simulink model "s_aero_2dof_lqr_control"  (R2017a)
settings: Solver=ode1  StartTime=0.0  StopTime=30  FixedStep=0.002  RelTol=1e-3  EnableMultiTasking=on
values from neighbouring files (symbols this model uses):
  K = lqr(A,B,Q,R)    [quanser_aero_lqr.m]    (also in quanser_aero_pd_design.m = Kyy/Dy)
undefined symbols (not defined in the file or in its folder): A, B, C, D
libraries: simulink_extras x4, quarc_library x2
settings Model: ExtModeTrigDuration=5000  Creator=MLevis  LastModifiedBy=Administrator
settings SolverCC: PositivePriorityOrder=on
settings DataIOCC: LimitDataPoints=on  SaveFormat=Array
settings OptimizationCC: LifeSpan=inf
settings DebuggingCC: SolverPrmCheckMsg=warning  SFUnexpectedBacktrackingDiag=warning  SFNoUnconditionalDefaultTransitionDiag=warning  SFExecutionAtInitializationDiag=none
settings HardwareCC: ProdBitPerPointer=32  ProdBitPerSizeT=32  ProdBitPerPtrDiffT=32  ProdLargestAtomicFloat=None  ProdIntDivRoundTo=Undefined  ProdEndianess=Unspecified  ProdWordSize=32  ProdHWDeviceType=32-bit Generic
settings ModelReferenceCC: PropagateSignalLabelsOutOfModel=off
settings RTWCC: SystemTargetFile=quarc_win64.tlc  TemplateMakefile=quarc_default_tmf  Description=QUARC Win64 Target
settings STFCustomTargetCC: TargetPreCompLibLocation=C:\PROGRA~3\QUARC\lib\2014a\win64\release  ConcurrentExecutionCompliant=on  GeneratePreprocessorConditionals=Disable all  SystemTargetFile=quarc_win64.tlc
settings GRTTargetCC: TargetPreCompLibLocation=C:\PROGRA~3\QUARC\lib\2014a\win64\release  TargetLangStandard=C89/C90 (ANSI)  ParMdlRefBuildCompliant=off  CompOptLevelCompliant=off  GeneratePreprocessorConditionals=Disable all  CombineOutputUpdateFcns=off  MatFileLogging=off  CPPClassGenCompliant=off  GRTInterface=on  UseToolchainInfoCompliant=off  ExtMode=on  ExtModeMexFile=quarc_comm
settings ConfigComp: CovMetricSettings=dw  CovHtmlReporting=on  CovSaveCumulativeToWorkspaceVar=on  CovSaveSingleToWorkspaceVar=on  CovExternalEMLEnable=off  CovSFcnEnable=off

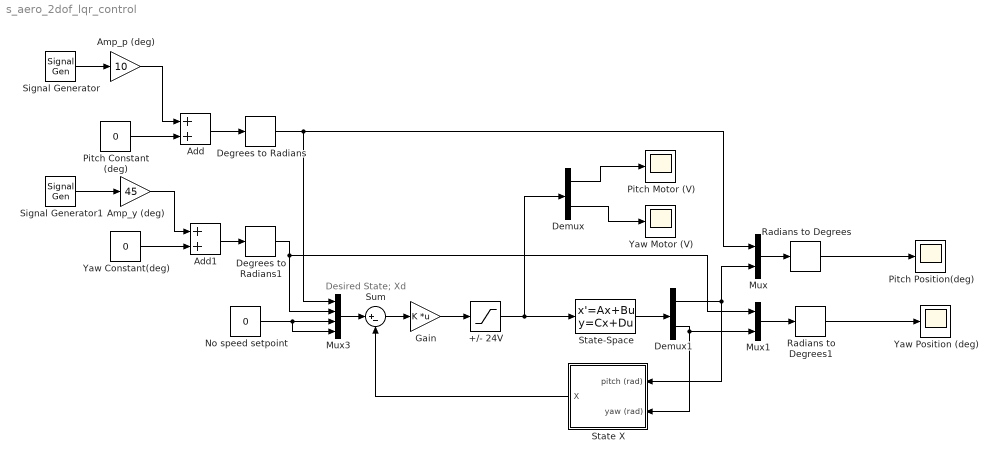
== system s_aero_2dof_lqr_control ==
  note: Desired State; Xd
  +/- 24V : Saturate  UpperLimit=24  LowerLimit=-24
  Add : Sum
  Add1 : Sum
  Amp_p (deg) : Gain  Gain=10
  Amp_y (deg) : Gain  Gain=45
  Degrees to Radians : simulink_extras/Transformations/Degrees to Radians
  Degrees to Radians1 : simulink_extras/Transformations/Degrees to Radians
  Demux : Demux  Outputs=2
  Demux1 : Demux  Outputs=2
  Gain : Gain  Gain=K  Multiplication=Matrix(K*u)
  Mux : Mux  Inputs=2
  Mux1 : Mux  Inputs=2
  Mux3 : Mux
  No speed setpoint : Constant  Value=0
  Pitch Constant (deg) : Constant  Value=0
  Pitch Motor (V) : Scope
  Pitch Position(deg) : Scope
  Radians to Degrees : simulink_extras/Transformations/Radians to Degrees
  Radians to Degrees1 : simulink_extras/Transformations/Radians to Degrees
  Signal Generator : SignalGenerator  WaveForm=square  Frequency=0.1
  Signal Generator1 : SignalGenerator  WaveForm=square  Frequency=0.04
  State X : Subsystem
  State-Space : StateSpace  A=A  B=B  C=C  D=D  X0=0
  Sum : Sum  Inputs=|+-
  Yaw Constant(deg) : Constant  Value=0
  Yaw Motor (V) : Scope
  Yaw Position (deg) : Scope
  wires:
  Degrees to Radians/1 -> Mux3/1, Mux/1
  Degrees to Radians1/1 -> Mux3/2, Mux1/1
  Signal Generator/1 -> Amp_p (deg)/1
  Pitch Constant (deg)/1 -> Add/2
  Add/1 -> Degrees to Radians/1
  Yaw Constant(deg)/1 -> Add1/2
  Amp_p (deg)/1 -> Add/1
  Signal Generator1/1 -> Amp_y (deg)/1
  Amp_y (deg)/1 -> Add1/1
  Add1/1 -> Degrees to Radians1/1
  Mux/1 -> Radians to Degrees/1
  Radians to Degrees/1 -> Pitch Position(deg)/1
  Radians to Degrees1/1 -> Yaw Position (deg)/1
  Gain/1 -> +/- 24V/1
  Demux/1 -> Pitch Motor (V)/1
  Demux/2 -> Yaw Motor (V)/1
  Sum/1 -> Gain/1
  Mux1/1 -> Radians to Degrees1/1
  Mux3/1 -> Sum/1
  No speed setpoint/1 -> Mux3/4, Mux3/3
  +/- 24V/1 -> State-Space/1, Demux/1
  State X/1(X) -> Sum/2
  Demux1/1 -> Mux/2, State X/1(pitch (rad))
  State-Space/1 -> Demux1/1
  Demux1/2 -> Mux1/2, State X/2(yaw (rad))

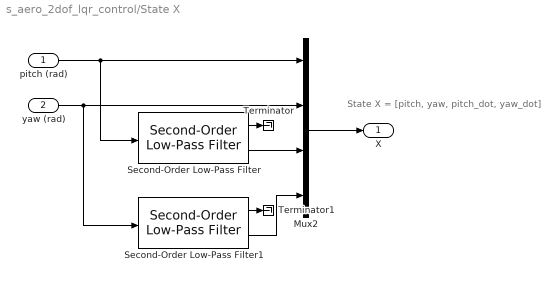
== system s_aero_2dof_lqr_control/State X ==
  note: State X = [pitch, yaw, pitch_dot, yaw_dot]
  pitch (rad) : Inport
  yaw (rad) : Inport  Port=2
  Mux2 : Mux
  Second-Order Low-Pass Filter : quarc_library/Continuous/Second-Order Low-Pass Filter  params_source=Internal (dialog parameters)  input_width=50  input_zeta=0.8  input_init=0
  Second-Order Low-Pass Filter1 : quarc_library/Continuous/Second-Order Low-Pass Filter  params_source=Internal (dialog parameters)  input_width=50  input_zeta=0.8  input_init=0
  Terminator : Terminator
  Terminator1 : Terminator
  X : Outport
  wires:
  Mux2/1 -> X/1
  yaw (rad)/1 -> Second-Order Low-Pass Filter1/1, Mux2/2
  pitch (rad)/1 -> Second-Order Low-Pass Filter/1, Mux2/1
  Second-Order Low-Pass Filter/2 -> Mux2/3
  Second-Order Low-Pass Filter1/2 -> Mux2/4
  Second-Order Low-Pass Filter/1 -> Terminator/1
  Second-Order Low-Pass Filter1/1 -> Terminator1/1
